simulink model "MSFartoystyring_1_8_new"  (R2018a)
settings: Solver=ode45  StartTime=tstart  StopTime=tstop  RelTol=1e-3  EnableMultiTasking=on
values from neighbouring files (symbols this model uses):
  c = 1    [run.m]    (also in run_2.m; run_task_1_4.m = 0; run_task_1_6.m = 0; run_task_1_6_new.m = 0)
  d_1 = D(1)    [run_task_1_6_new.m]
  d_2 = D(2)    [run_task_1_6_new.m]
  dc_max = 25*(pi/180)    (= 0.436332312999)    [run_task_1_8.m]
  kd_heading = 2*zeta*omegan*(m+km)-d    [run_2.m]    (also in run_task_1_7.m = 0; run_task_1_8.m)
  ki_heading = omegan/10*kp_heading    [run_2.m]    (also in run_task_1_7.m; run_task_1_8.m)
  ki_surge = 0    [run_2.m]    (also in run_task_1_7.m; run_task_1_8.m)
  kp_heading = (m+km)*omegan^2-k    [run_2.m]    (also in run_task_1_7.m; run_task_1_8.m)
  kp_surge = 100    [run_2.m]    (also in run_task_1_7.m = 5; run_task_1_8.m)
  m_u = 5500    [run_task_1_6_new.m]
  nc_max = (85*2*pi)/60    (= 8.90117918517)    [run.m]    (also in run_2.m; run_task_1_7.m; run_task_1_8.m)
  p0 = zeros(2,1)    [run.m]    (also in run_2.m = [1000 700]'; run_task_1_4.m; run_task_1_6.m; run_task_1_6_new.m)
  psi0 = 0    [run.m]    (also in run_2.m; run_task_1_4.m; run_task_1_6.m; run_task_1_6_new.m)
  r0 = 0    [run.m]    (also in run_2.m; run_task_1_4.m; run_task_1_6.m; run_task_1_6_new.m)
  tsamp = 10    [run.m]    (also in run_2.m; run_task_1_4.m; run_task_1_6.m; run_task_1_6_new.m)
  v0 = [3 0]'    [run.m]    (also in run_2.m = [6.63 0]'; run_task_1_4.m = [6.63 0]'; run_task_1_6.m = [0.001 0]'; run_task_1_6_new.m = [0.001 0]')
  zeta_surge = 1.2    [run_2.m]    (also in run_task_1_8.m)
undefined symbols (not defined in the file or in its folder): msfartoystyring, omega_surge, sgn, u_r_0
settings Model: ExtModeAutoUpdateStatusClock=off  Creator=christh  LastModifiedBy=sondr
settings SolverCC: AlgebraicLoopSolver=LineSearch
settings DataIOCC: LimitDataPoints=on  SaveFormat=Array  SignalLoggingSaveFormat=ModelDataLogs
settings OptimizationCC: ExpressionDepthLimit=2147483647  InitFltsAndDblsToZero=on  LifeSpan=inf
settings DebuggingCC: UnderspecifiedInitializationDetection=Classic  MergeDetectMultiDrivingBlocksExec=none  SolverPrmCheckMsg=warning  FcnCallInpInsideContextMsg=warning  StateNameClashWarn=warning  SFUnexpectedBacktrackingDiag=warning  SFNoUnconditionalDefaultTransitionDiag=warning  SFExecutionAtInitializationDiag=none
settings HardwareCC: ProdBitPerPointer=32  ProdBitPerSizeT=32  ProdBitPerPtrDiffT=32  ProdLargestAtomicFloat=None  ProdIntDivRoundTo=Undefined  ProdEndianess=Unspecified  ProdWordSize=32  ProdHWDeviceType=32-bit Generic
settings ModelReferenceCC: PropagateSignalLabelsOutOfModel=off
settings CodeAppCC: StateflowObjectComments=on
settings GRTTargetCC: TargetLangStandard=C89/C90 (ANSI)  GeneratePreprocessorConditionals=Disable all  CombineOutputUpdateFcns=off  GRTInterface=on
settings ConfigComp: CovMetricSettings=dw  CovHtmlReporting=on  CovSaveCumulativeToWorkspaceVar=on  CovSaveSingleToWorkspaceVar=on  CovExternalEMLEnable=off

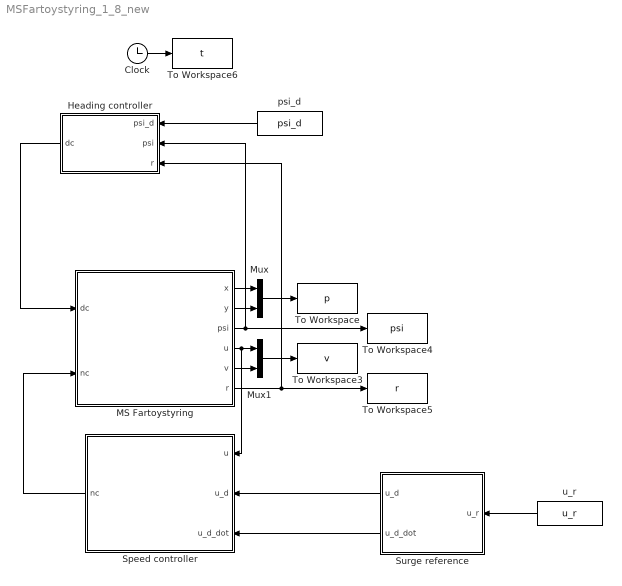
== system MSFartoystyring_1_8_new ==
  Clock : Clock
  Heading controller : Subsystem
  MS Fartoystyring : Subsystem  mask(MS Fartoystyring for Assignment 3 G&C){x0=p0(1), y0=p0(2), u0=v0(1), v0=v0(2), psi0=psi0, r0=r0, c=c}
      mask prompts: x0 "x(t0) (m)"; y0 "y(t0) (m)"; u0 "u(t0) (m/s)"; v0 "v(t0) (m/s)"; psi0 "psi(t0) (rad)"; r0 "r(t0) (rad/s)"; c "current (0 or 1)"
      mask help:
      | Block corresponding to Figure 1 in the assignment text. Gives the response of the ship.
      |
      | The design speed of MS Fartoystyring is u=8.23 m/s.
      |
      | Input:
      | dc: commanded rudder (rad), dmax=25*pi/180
      | nc: commanded shaft speed (rad/s), nmax=85*2*pi/60
      |
      | Output:
      | x: north pos (m)
      | y: east pos (m)
      | u: surge (m/s)
      | v: sway (m/s)
      | psi: heading (rad)
      | r: yaw (rad/s)
      mask Help: Comments, bugs and help requests can be directed to the TA. Email on course website.
  Mux : Mux  Inputs=2
  Mux1 : Mux  Inputs=2
  "Speed controller " : Subsystem
  Surge reference : Subsystem
  To Workspace : ToWorkspace  VariableName=p  SampleTime=tsamp
  To Workspace3 : ToWorkspace  VariableName=v  SampleTime=tsamp
  To Workspace4 : ToWorkspace  VariableName=psi  SampleTime=tsamp
  To Workspace5 : ToWorkspace  VariableName=r  SampleTime=tsamp
  To Workspace6 : ToWorkspace  VariableName=t  SampleTime=tsamp
  psi_d : FromWorkspace  VariableName=psi_d  SampleTime=0
  u_r : FromWorkspace  VariableName=u_r  SampleTime=0
  wires:
  Clock/1 -> To Workspace6/1
  MS Fartoystyring/1(x) -> Mux/1
  MS Fartoystyring/2(y) -> Mux/2
  MS Fartoystyring/4(u) -> "Speed controller "/1(u), Mux1/1
  MS Fartoystyring/5(v) -> Mux1/2
  Mux/1 -> To Workspace/1
  Mux1/1 -> To Workspace3/1
  MS Fartoystyring/3(psi) -> Heading controller/2("psi "), To Workspace4/1
  MS Fartoystyring/6(r) -> Heading controller/3("r "), To Workspace5/1
  Heading controller/1("dc ") -> MS Fartoystyring/1(dc)
  psi_d/1 -> Heading controller/1(psi_d)
  "Speed controller "/1(nc) -> MS Fartoystyring/2(nc)
  Surge reference/1(u_d) -> "Speed controller "/2(u_d)
  u_r/1 -> Surge reference/1(u_r)
  Surge reference/2(u_d_dot) -> "Speed controller "/3(u_d_dot)

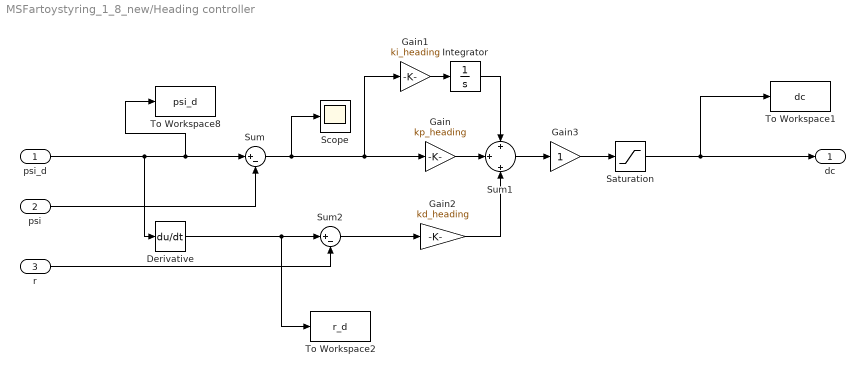
== system MSFartoystyring_1_8_new/Heading controller ==
  psi_d : Inport
  "psi " : Inport  Port=2
  "r " : Inport  Port=3
  Derivative : Derivative
  Gain : Gain  Gain=kp_heading
  Gain1 : Gain  Gain=ki_heading
  Gain2 : Gain  Gain=kd_heading
  Gain3 : Gain
  Integrator : Integrator
  Saturation : Saturate  UpperLimit=dc_max  LowerLimit=-dc_max
  Scope : Scope
  Sum : Sum  Inputs=|+-
  Sum1 : Sum  Inputs=+|+|+
  Sum2 : Sum  Inputs=|+-
  To Workspace1 : ToWorkspace  VariableName=dc  SampleTime=tsamp
  To Workspace2 : ToWorkspace  VariableName=r_d  SampleTime=tsamp
  To Workspace8 : ToWorkspace  VariableName=psi_d  SampleTime=tsamp
  "dc " : Outport
  wires:
  Sum/1 -> Scope/1, Gain/1, Gain1/1
  Gain1/1 -> Integrator/1
  Sum1/1 -> Gain3/1
  Gain/1 -> Sum1/2
  Gain2/1 -> Sum1/3
  Gain3/1 -> Saturation/1
  Integrator/1 -> Sum1/1
  "psi "/1 -> Sum/2
  Derivative/1 -> To Workspace2/1, Sum2/1
  psi_d/1 -> To Workspace8/1, Sum/1, Derivative/1
  Sum2/1 -> Gain2/1
  "r "/1 -> Sum2/2
  Saturation/1 -> To Workspace1/1, "dc "/1

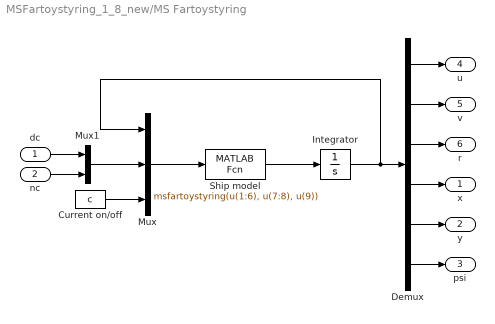
== system MSFartoystyring_1_8_new/MS Fartoystyring ==
  dc : Inport
  nc : Inport  Port=2
  Current on/off : Constant  Value=c
  Demux : Demux  Outputs=6
  Integrator : Integrator  InitialCondition=[u0 v0 r0 x0 y0 psi0]'
  Mux : Mux  Inputs=3
  Mux1 : Mux  Inputs=2
  Ship model : MATLABFcn  MATLABFcn=msfartoystyring(u(1:6), u(7:8), u(9))  OutputDimensions=6
  x : Outport
  y : Outport  Port=2
  psi : Outport  Port=3
  u : Outport  Port=4
  v : Outport  Port=5
  r : Outport  Port=6
  wires:
  Integrator/1 -> Mux/1, Demux/1
  Mux1/1 -> Mux/2
  dc/1 -> Mux1/1
  nc/1 -> Mux1/2
  Demux/1 -> u/1
  Demux/2 -> v/1
  Demux/3 -> r/1
  Demux/4 -> x/1
  Demux/5 -> y/1
  Demux/6 -> psi/1
  Current on/off/1 -> Mux/3
  Ship model/1 -> Integrator/1
  Mux/1 -> Ship model/1

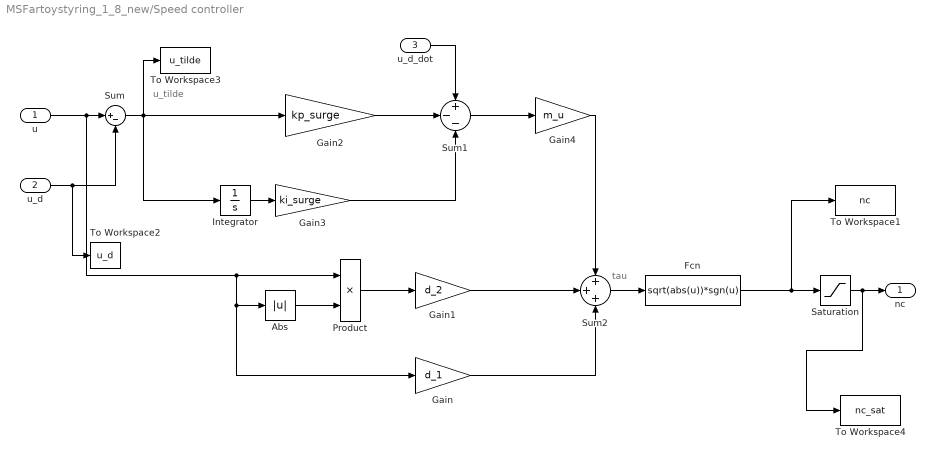
== system MSFartoystyring_1_8_new/Speed controller  ==
  note: tau
  note: u_tilde
  u : Inport
  u_d : Inport  Port=2
  u_d_dot : Inport  Port=3
  Abs : Abs
  Fcn : Fcn  Expr=sqrt(abs(u))*sgn(u)
  Gain : Gain  Gain=d_1
  Gain1 : Gain  Gain=d_2
  Gain2 : Gain  Gain=kp_surge
  Gain3 : Gain  Gain=ki_surge
  Gain4 : Gain  Gain=m_u
  Integrator : Integrator
  Product : Product
  Saturation : Saturate  UpperLimit=nc_max  LowerLimit=0
  Sum : Sum  Inputs=|+-
  Sum1 : Sum  Inputs=+--
  Sum2 : Sum  Inputs=+++
  To Workspace1 : ToWorkspace  VariableName=nc  SampleTime=tsamp
  To Workspace2 : ToWorkspace  VariableName=u_d  SampleTime=tsamp
  To Workspace3 : ToWorkspace  VariableName=u_tilde  SampleTime=tsamp
  To Workspace4 : ToWorkspace  VariableName=nc_sat  SampleTime=tsamp
  nc : Outport
  wires:
  u/1 -> Abs/1, Gain/1, Product/1, Sum/1
  u_d/1 -> To Workspace2/1, Sum/2
  Sum/1 -> Gain2/1, Integrator/1, To Workspace3/1
  Gain2/1 -> Sum1/2
  u_d_dot/1 -> Sum1/1
  Sum1/1 -> Gain4/1
  Gain4/1 -> Sum2/1
  Sum2/1 -> Fcn/1
  Gain1/1 -> Sum2/2
  Product/1 -> Gain1/1
  Abs/1 -> Product/2
  Gain/1 -> Sum2/3
  Gain3/1 -> Sum1/3
  Fcn/1 -> Saturation/1, To Workspace1/1
  Saturation/1 -> To Workspace4/1, nc/1
  Integrator/1 -> Gain3/1

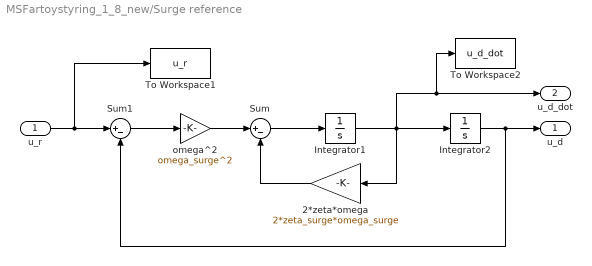
== system MSFartoystyring_1_8_new/Surge reference ==
  u_r : Inport
  2*zeta*omega : Gain  Gain=2*zeta_surge*omega_surge
  Integrator1 : Integrator
  Integrator2 : Integrator  InitialCondition=u_r_0
  Sum : Sum  Inputs=|+-
  Sum1 : Sum  Inputs=|+-
  To Workspace1 : ToWorkspace  VariableName=u_r  SampleTime=tsamp
  To Workspace2 : ToWorkspace  VariableName=u_d_dot  SampleTime=tsamp
  omega^2 : Gain  Gain=omega_surge^2
  u_d : Outport
  u_d_dot : Outport  Port=2
  wires:
  Sum/1 -> Integrator1/1
  Integrator1/1 -> 2*zeta*omega/1, To Workspace2/1, u_d_dot/1, Integrator2/1
  omega^2/1 -> Sum/1
  2*zeta*omega/1 -> Sum/2
  u_r/1 -> Sum1/1, To Workspace1/1
  Sum1/1 -> omega^2/1
  Integrator2/1 -> Sum1/2, u_d/1
